simulink model "Model_test - 副本 (2)"  (R2022b)
settings: Solver=VariableStepAuto  StartTime=0.0  StopTime=10.0  RelTol=1e-3
settings Model: Creator=wukang  LastModifiedBy=wukang

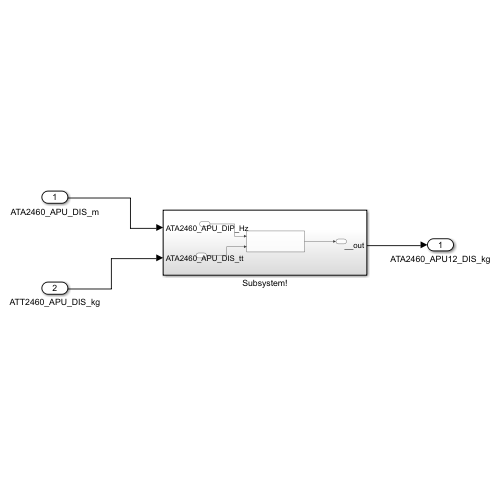
[thumbnail: Simulink's stored preview of the top-level diagram]
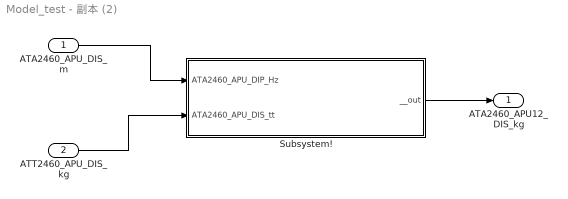
== system Model_test - 副本 (2) ==
  ATA2460_APU_DIS_m : Inport
  ATT2460_APU_DIS_kg : Inport  Port=2
  Subsystem! : Subsystem
  ATA2460_APU12_DIS_kg : Outport
  wires:
  ATA2460_APU_DIS_m/1 -> Subsystem!/1(ATA2460_APU_DIP_Hz)
  ATT2460_APU_DIS_kg/1 -> Subsystem!/2(ATA2460_APU_DIS_tt)
  Subsystem!/1(__out) -> ATA2460_APU12_DIS_kg/1

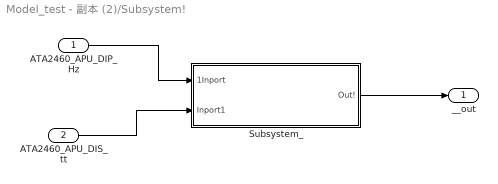
== system Model_test - 副本 (2)/Subsystem! ==
  ATA2460_APU_DIP_Hz : Inport
  ATA2460_APU_DIS_tt : Inport  Port=2
  Subsystem_ : Subsystem  mask{Parameter__1=0}
      mask DialogControl ParameterGroupVar Prompt: 参数
  __out : Outport
  wires:
  ATA2460_APU_DIS_tt/1 -> Subsystem_/2(" Inport1")
  Subsystem_/1(Out!) -> __out/1
  ATA2460_APU_DIP_Hz/1 -> Subsystem_/1(1Inport)

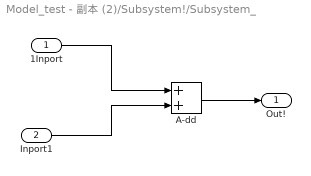
== system Model_test - 副本 (2)/Subsystem!/Subsystem_ ==
  1Inport : Inport
  " Inport1" : Inport  Port=2
  A-dd : Sum
  Out! : Outport
  wires:
  " Inport1"/1 -> A-dd/2
  1Inport/1 -> A-dd/1
  A-dd/1 -> Out!/1
